simulink model "HDLFixedPoint"  (R2024a)
settings: Solver=FixedStepDiscrete  StartTime=0.0  StopTime=stopTime  RelTol=1e-3
libraries: dspsrcs4 x2
settings Model: DataTypeOverride=Off  MinMaxOverflowLogging=ForceOff  FPTRunName=fxpOptimization.BaselineRun  SimulationMode=accelerator  Creator=cotti  LastModifiedBy=cotti
settings DataIOCC: SaveOutput=off  SaveTime=off
settings OptimizationCC: BlockReduction=off  ConditionallyExecuteInputs=off  DefaultParameterBehavior=Inlined  InheritOutputTypeSmallerThanSingle=on
settings DebuggingCC: SignalRangeChecking=error  AlgebraicLoopMsg=error  SingleTaskRateTransMsg=error  IntegerOverflowMsg=none  ParameterDowncastMsg=none  ParameterOverflowMsg=none  ParameterPrecisionLossMsg=none  UnconnectedInputMsg=warning  UnconnectedOutputMsg=warning  UnconnectedLineMsg=warning  IntegerSaturationMsg=none
settings HardwareCC: ProdBitPerPointer=32  ProdBitPerSizeT=32  ProdBitPerPtrDiffT=32  ProdLargestAtomicFloat=None  ProdIntDivRoundTo=Undefined  ProdEndianess=Unspecified  ProdWordSize=32  ProdHWDeviceType=ASIC/FPGA->ASIC/FPGA  TargetBitPerLong=64  TargetBitPerPointer=64  TargetBitPerSizeT=64  TargetBitPerPtrDiffT=64  TargetLongLongMode=on  TargetIntDivRoundTo=Zero  TargetEndianess=LittleEndian  TargetWordSize=64  TargetHWDeviceType=Custom Processor->MATLAB Host Computer  ProdEqTarget=off

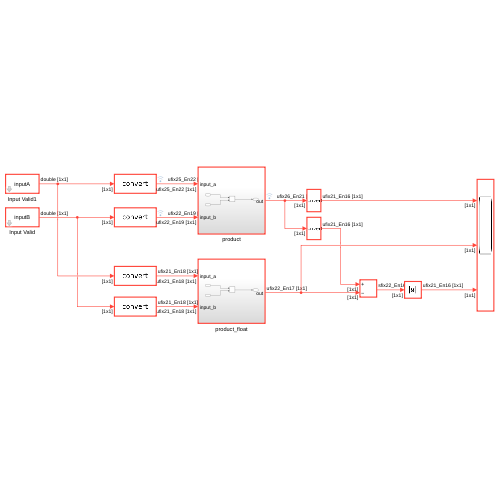
[thumbnail: Simulink's stored preview of the top-level diagram]
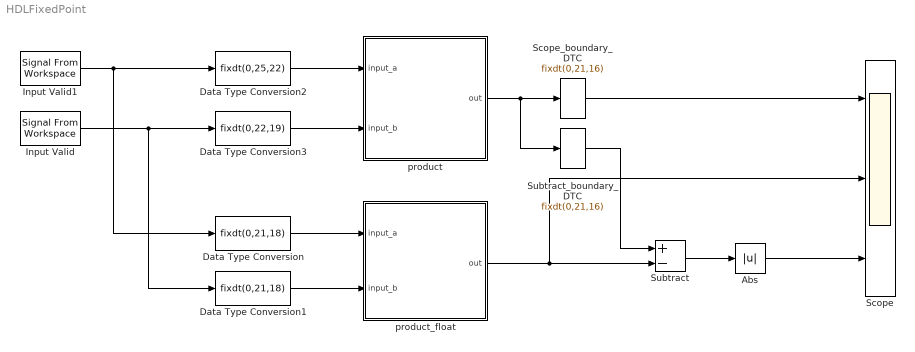
== system HDLFixedPoint ==
  Abs : Abs  OutDataTypeStr=fixdt(0,21,16)  SaturateOnIntegerOverflow=off
  Data Type Conversion : DataTypeConversion  OutDataTypeStr=fixdt(0,21,18)  SaturateOnIntegerOverflow=off  RndMeth=Floor
  Data Type Conversion1 : DataTypeConversion  OutDataTypeStr=fixdt(0,21,18)  SaturateOnIntegerOverflow=off  RndMeth=Floor
  Data Type Conversion2 : DataTypeConversion  OutMin=0  OutMax=5  OutDataTypeStr=fixdt(0,25,22)  SaturateOnIntegerOverflow=off  RndMeth=Floor
  Data Type Conversion3 : DataTypeConversion  OutMin=0  OutMax=5  OutDataTypeStr=fixdt(0,22,19)  SaturateOnIntegerOverflow=off  RndMeth=Floor
  Input Valid : dspsrcs4/Signal From Workspace  X=inputB  Ts=1  nsamps=1  OutputAfterFinalValue=Setting to zero  ignoreOrWarnInputAndFrameLengths=off  OutputFrames=off
  Input Valid1 : dspsrcs4/Signal From Workspace  X=inputA  Ts=1  nsamps=1  OutputAfterFinalValue=Setting to zero  ignoreOrWarnInputAndFrameLengths=off  OutputFrames=off
  Scope : Scope  NumInputPorts=3
  Scope_boundary_DTC : DataTypeConversion  OutDataTypeStr=fixdt(0,21,16)
  Subtract : Sum  Inputs=+-  OutDataTypeStr=fixdt(1,22,16)  AccumDataTypeStr=fixdt(1,22,15)
  Subtract_boundary_DTC : DataTypeConversion  OutDataTypeStr=fixdt(0,21,16)
  product : Subsystem
  product_float : Subsystem
  wires:
  product/1(out) -> Scope_boundary_DTC/1, Subtract_boundary_DTC/1
  Input Valid1/1 -> Data Type Conversion/1, Data Type Conversion2/1
  Input Valid/1 -> Data Type Conversion1/1, Data Type Conversion3/1
  Data Type Conversion/1 -> product_float/1(input_a)
  Data Type Conversion1/1 -> product_float/2(input_b)
  Data Type Conversion2/1 -> product/1(input_a)
  Data Type Conversion3/1 -> product/2(input_b)
  product_float/1(out) -> Subtract/2, Scope/2
  Subtract/1 -> Abs/1
  Abs/1 -> Scope/3
  Scope_boundary_DTC/1 -> Scope/1
  Subtract_boundary_DTC/1 -> Subtract/1

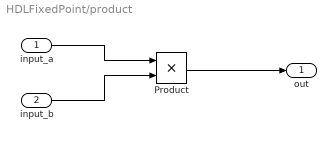
== system HDLFixedPoint/product ==
  input_a : Inport  OutDataTypeStr=fixdt(0,25,22)
  input_b : Inport  Port=2  OutDataTypeStr=fixdt(0,22,19)
  Product : Product  OutDataTypeStr=fixdt(0,26,21)
  out : Outport  OutDataTypeStr=fixdt(0,26,21)
  wires:
  input_a/1 -> Product/1
  input_b/1 -> Product/2
  Product/1 -> out/1

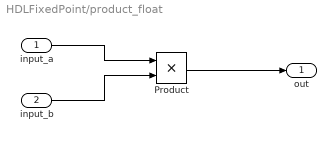
== system HDLFixedPoint/product_float ==
  input_a : Inport  OutDataTypeStr=fixdt(0,21,18)
  input_b : Inport  Port=2  OutDataTypeStr=fixdt(0,21,18)
  Product : Product  OutDataTypeStr=fixdt(0,22,17)
  out : Outport  OutDataTypeStr=fixdt(0,22,17)
  wires:
  input_a/1 -> Product/1
  input_b/1 -> Product/2
  Product/1 -> out/1
